simulink model "FaultDetection_Harness1"  (R2022b)
settings: configuration reference "BMS_Sw_CodeGenConfig" (kept outside this file)
settings Model: DataDictionary=Shared_DD.sldd  Creator=cpatel  LastModifiedBy=cpatel
settings ConfigSetRef: SourceName=BMS_Sw_CodeGenConfig

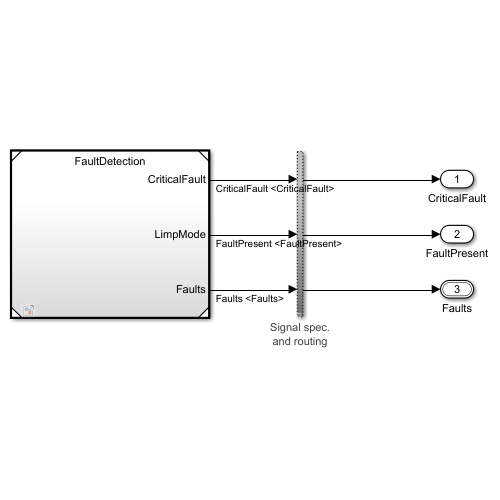
[thumbnail: Simulink's stored preview of the top-level diagram]
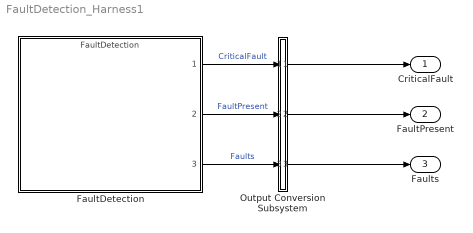
== system FaultDetection_Harness1 ==
  FaultDetection : ModelReference  ModelNameDialog=FaultDetection  SimulationMode=Normal  ModelReferenceVersion=5.25
  Output Conversion Subsystem : Subsystem  Tag=__SLT_OCS__  Description=|
      | Signal spec.
      | and routing
      settings: AttributesFormatString=%<Description>
  CriticalFault : Outport
  FaultPresent : Outport  Port=2
  Faults : Outport  Port=3  OutDataTypeStr=Bus: Faults
  wires:
  FaultDetection/1 -> Output Conversion Subsystem/1(Inport_1)  "CriticalFault"
  FaultDetection/2 -> Output Conversion Subsystem/2(Inport_2)  "FaultPresent"
  FaultDetection/3 -> Output Conversion Subsystem/3(Inport_3)  "Faults"
  Output Conversion Subsystem/3(Outport_3) -> Faults/1
  Output Conversion Subsystem/2(Outport_2) -> FaultPresent/1
  Output Conversion Subsystem/1(Outport_1) -> CriticalFault/1

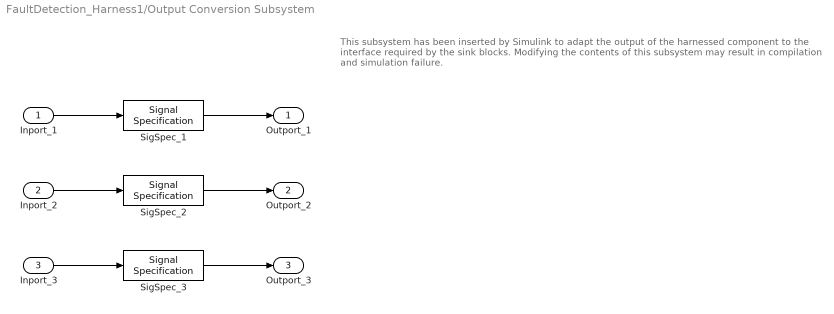
== system FaultDetection_Harness1/Output Conversion Subsystem ==
  note: This subsystem has been inserted by Simulink to adapt the output of the harnessed component to the interface required by the sink blocks.
      |  Modifying the contents of this subsystem may result in compilation and simulation failure.
  Inport_1 : Inport
  Inport_2 : Inport  Port=2
  Inport_3 : Inport  Port=3
  SigSpec_1 : SignalSpecification  OutDataTypeStr=boolean  Dimensions=[1]  SampleTime=180
  SigSpec_2 : SignalSpecification  OutDataTypeStr=boolean  Dimensions=[1]  SampleTime=180
  SigSpec_3 : SignalSpecification  OutDataTypeStr=Bus: Faults  Dimensions=[1]  SampleTime=180  BusOutputAsStruct=on
  Outport_1 : Outport
  Outport_2 : Outport  Port=2
  Outport_3 : Outport  Port=3
  wires:
  Inport_1/1 -> SigSpec_1/1
  SigSpec_1/1 -> Outport_1/1
  Inport_2/1 -> SigSpec_2/1
  SigSpec_2/1 -> Outport_2/1
  Inport_3/1 -> SigSpec_3/1
  SigSpec_3/1 -> Outport_3/1
